simulink library "HysteresisFilterBlock"  (R2018b)
settings: Solver=VariableStepAuto  StartTime=0.0  StopTime=10.0  RelTol=1e-3
undefined symbols (not defined in the file): signal_hold_time
libraries: simulink x2
settings Model: Creator=BI28030  LastModifiedBy=BI28030

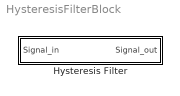
== system HysteresisFilterBlock ==
  Hysteresis Filter : Subsystem  mask(Filter Signal){signal_hold_time=signal_hold_time}
      mask prompts: signal_hold_time "Signal Hold Time (s)"
      mask help: Holds signal level for at least the specified time unless the signal level increases.

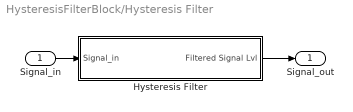
== system HysteresisFilterBlock/Hysteresis Filter ==
  Signal_in : Inport
  Hysteresis Filter : Subsystem
  Signal_out : Outport
  wires:
  Signal_in/1 -> Hysteresis Filter/1(Signal_in)
  Hysteresis Filter/1(Filtered Signal Lvl) -> Signal_out/1

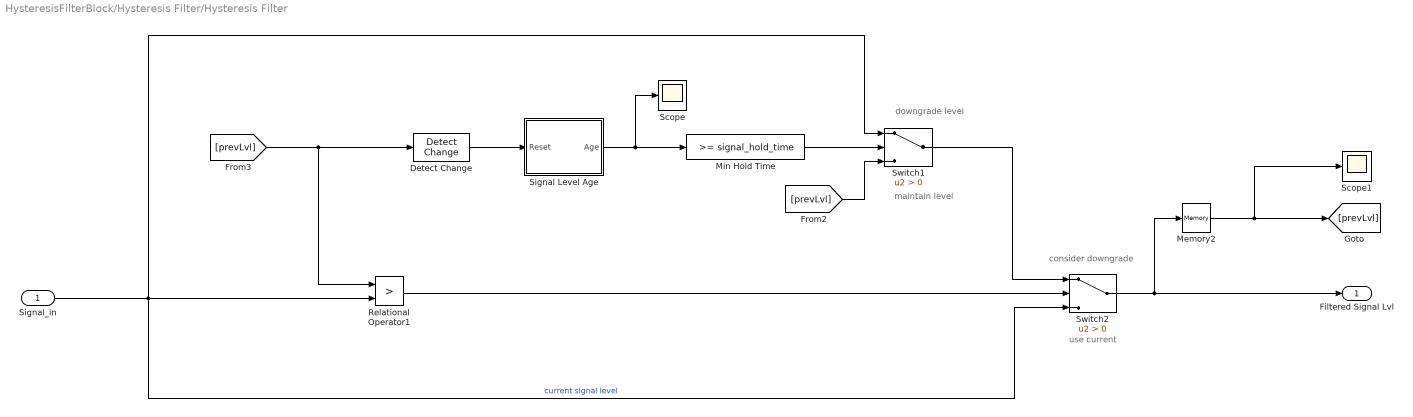
== system HysteresisFilterBlock/Hysteresis Filter/Hysteresis Filter ==
  note: downgrade level
  note: maintain level
  note: consider downgrade
  note: use current
  Signal_in : Inport
  Detect Change : simulink/Logic and Bit Operations/Detect Change  vinit=0  OutDataTypeStr=boolean
  Memory2 : Memory  InheritSampleTime=on
  Min Hold Time : simulink/Logic and Bit Operations/Compare To Constant  relop=>=  const=signal_hold_time  OutDataTypeStr=boolean
  Relational Operator1 : RelationalOperator  Operator=>  OutDataTypeStr=boolean  RndMeth=Nearest
  Scope : Scope
  Scope1 : Scope
  Signal Level Age : Subsystem
  Switch1 : Switch  Criteria=u2 > Threshold
  Switch2 : Switch  Criteria=u2 > Threshold
  Filtered Signal Lvl : Outport
  wires:
  Detect Change/1 -> Signal Level Age/1(Reset)
  [prevLvl] -> Detect Change/1, Relational Operator1/1
  Relational Operator1/1 -> Switch2/2
  Signal Level Age/1(Age) -> Min Hold Time/1, Scope/1
  [prevLvl] -> Switch1/3
  Memory2/1 -> Scope1/1, [prevLvl]
  Signal_in/1 -> Switch2/3, Relational Operator1/2, Switch1/1  "current signal level"
  Switch2/1 -> Filtered Signal Lvl/1, Memory2/1
  Switch1/1 -> Switch2/1
  Min Hold Time/1 -> Switch1/2

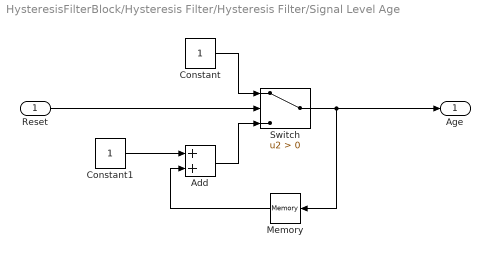
== system HysteresisFilterBlock/Hysteresis Filter/Hysteresis Filter/Signal Level Age ==
  Reset : Inport
  Add : Sum
  Constant : Constant
  Constant1 : Constant
  Memory : Memory  InheritSampleTime=on
  Switch : Switch  Criteria=u2 > Threshold
  Age : Outport
  wires:
  Memory/1 -> Add/2
  Constant/1 -> Switch/1
  Switch/1 -> Memory/1, Age/1
  Constant1/1 -> Add/1
  Reset/1 -> Switch/2
  Add/1 -> Switch/3
